simulink model "INTER_IIT_2ndorder_with_noise_BEFORE_INTEGRATOR_DSM"  (R2024a)
settings: Solver=VariableStepAuto  StartTime=0.0  StopTime=1.085  RelTol=1e-3
undefined symbols (not defined in the file): DiscIntNeverNeededParam
libraries: dspsrcs4 x3
settings Model: Creator=somya  LastModifiedBy=shrey

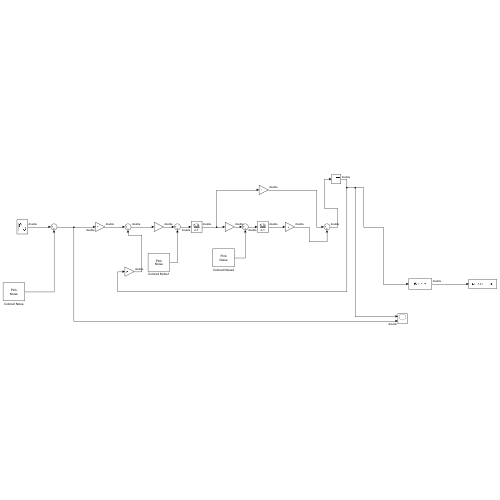
[thumbnail: Simulink's stored preview of the top-level diagram]
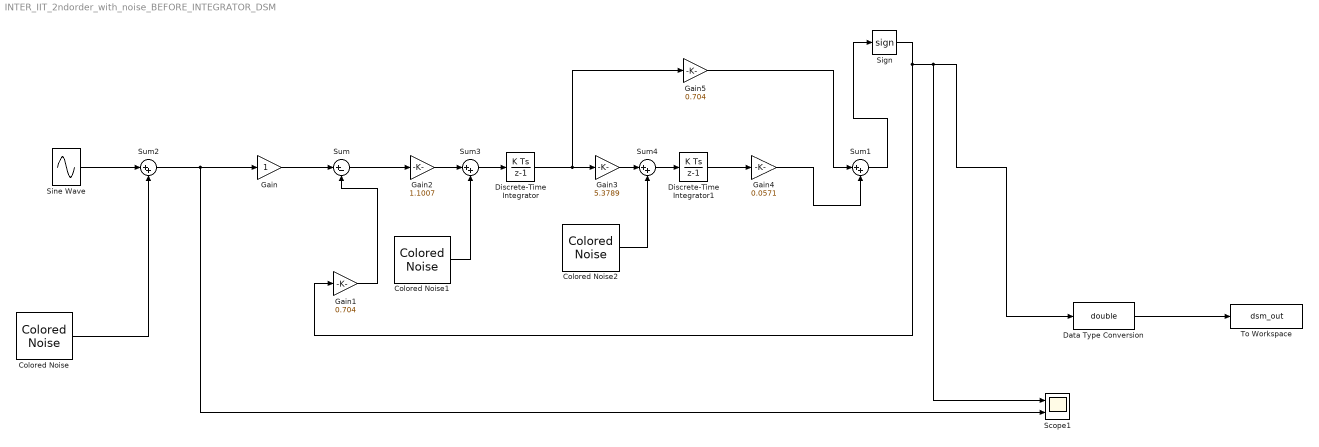
== system INTER_IIT_2ndorder_with_noise_BEFORE_INTEGRATOR_DSM ==
  Colored Noise : dspsrcs4/Colored Noise  Color=pink  InverseFrequencyPower=1  BoundedOutput=off  NumChannels=1  OutputDataType=double  SamplesPerFrame=1  SampleTime=1000  RandomStream=mt19937ar with seed  Seed=67  SimulateUsing=Interpreted execution
  Colored Noise1 : dspsrcs4/Colored Noise  Color=pink  InverseFrequencyPower=1  BoundedOutput=off  NumChannels=1  OutputDataType=double  SamplesPerFrame=1  SampleTime=1000  RandomStream=mt19937ar with seed  Seed=67  SimulateUsing=Interpreted execution
  Colored Noise2 : dspsrcs4/Colored Noise  Color=pink  InverseFrequencyPower=1  BoundedOutput=off  NumChannels=1  OutputDataType=double  SamplesPerFrame=1  SampleTime=1000  RandomStream=mt19937ar with seed  Seed=67  SimulateUsing=Interpreted execution
  Data Type Conversion : DataTypeConversion  OutDataTypeStr=double  SaturateOnIntegerOverflow=off  RndMeth=Floor
  Discrete-Time Integrator : DiscreteIntegrator  SampleTime=-1  ICPrevOutput=DiscIntNeverNeededParam  ICPrevScaledInput=DiscIntNeverNeededParam
  Discrete-Time Integrator1 : DiscreteIntegrator  SampleTime=-1  ICPrevOutput=DiscIntNeverNeededParam  ICPrevScaledInput=DiscIntNeverNeededParam
  Gain : Gain
  Gain1 : Gain  Gain=0.704
  Gain2 : Gain  Gain=1.1007
  Gain3 : Gain  Gain=5.3789
  Gain4 : Gain  Gain=0.0571
  Gain5 : Gain  Gain=0.704
  Scope1 : Scope  NumInputPorts=2
  Sign : Signum
  Sine Wave : Sin  Amplitude=0.5  Frequency=306.796157  Samples=150000  SampleTime=1.22e-7  VectorParams1D=off
  Sum : Sum  Inputs=|+-
  Sum{1..4} (4 alike) : Sum  Inputs=|++
  To Workspace : ToWorkspace  VariableName=dsm_out  SampleTime=-1
  wires:
  Gain/1 -> Sum/1
  Sum/1 -> Gain2/1
  Discrete-Time Integrator/1 -> Gain5/1, Gain3/1
  Gain5/1 -> Sum1/1
  Gain4/1 -> Sum1/2
  Sum1/1 -> Sign/1
  Gain1/1 -> Sum/2
  Discrete-Time Integrator1/1 -> Gain4/1
  Sign/1 -> Scope1/1, Data Type Conversion/1, Gain1/1
  Data Type Conversion/1 -> To Workspace/1
  Colored Noise/1 -> Sum2/2
  Sine Wave/1 -> Sum2/1
  Sum2/1 -> Scope1/2, Gain/1
  Gain2/1 -> Sum3/1
  Sum3/1 -> Discrete-Time Integrator/1
  Colored Noise1/1 -> Sum3/2
  Gain3/1 -> Sum4/1
  Sum4/1 -> Discrete-Time Integrator1/1
  Colored Noise2/1 -> Sum4/2
